simulink model "SixDOF_FlatEarth"  (R2018a)
settings: Solver=ode4  StartTime=0.0  StopTime=10  FixedStep=0.01  RelTol=1e-3
libraries: shared6dof x1, simulink x1
settings Model: Creator=Trajectories  LastModifiedBy=Trajectories

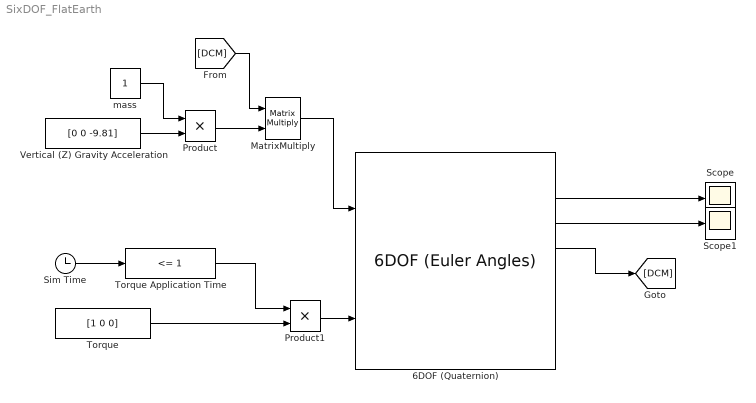
== system SixDOF_FlatEarth ==
  6DOF (Quaternion) : shared6dof/6DOF (Euler Angles)  units=Metric (MKS)  mtype=Fixed  rep=Quaternion  xme_0=[0 0 0]  Vm_0=[0 0 0]  eul_0=[0 0 0]  pm_0=[0 0 0]  mass_0=1.0  mass_e=0.5  mass_f=2.0  inertia=[10 0 0; 0 10 0; 0 0 10]  inertia_e=eye(3)  inertia_f=2*eye(3)  k_quat=1.0  vre_flag=on  abi_flag=off  aMode=0
      settings: SourceProductBaseCode=AE
  MatrixMultiply : Product  Multiplication=Matrix(*)
  Product : Product
  Product1 : Product
  Scope : Scope
  Scope1 : Scope
  Sim Time : Clock
  Torque : Constant  Value=[1 0 0]
  Torque Application Time : simulink/Logic and Bit Operations/Compare To Constant  relop=<=  const=1  OutDataTypeStr=boolean
  Vertical (Z) Gravity Acceleration : Constant  Value=[0 0 -9.81]
  mass : Constant
  wires:
  Vertical (Z) Gravity Acceleration/1 -> Product/2
  mass/1 -> Product/1
  Product/1 -> MatrixMultiply/2
  Sim Time/1 -> Torque Application Time/1
  Torque Application Time/1 -> Product1/1
  Torque/1 -> Product1/2
  Product1/1 -> 6DOF (Quaternion)/2
  6DOF (Quaternion)/2 -> Scope/1
  6DOF (Quaternion)/3 -> Scope1/1
  6DOF (Quaternion)/4 -> [DCM]
  [DCM] -> MatrixMultiply/1
  MatrixMultiply/1 -> 6DOF (Quaternion)/1
